simulink subsystem "startNormEcef2Body"  (R2021a)
settings: Solver=VariableStepAuto  StartTime=0.0  StopTime=10.0  RelTol=1e-3
libraries: dspmathops x1, sharedtransform x1
settings Model: Creator=noraw  LastModifiedBy=noraw

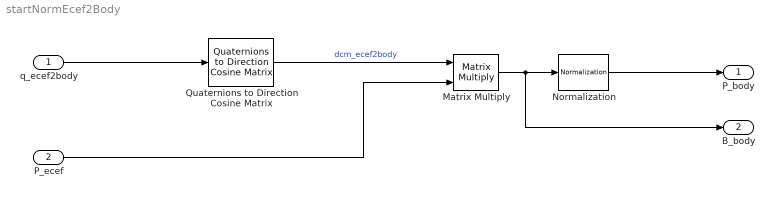
== system startNormEcef2Body ==
  q_ecef2body : Inport  PortDimensions=4
  P_ecef : Inport  Port=2  PortDimensions=3
  Matrix Multiply : Product  Multiplication=Matrix(*)
  Normalization : dspmathops/Normalization  NormType=2-norm  Bias=1e-10  NormOver=Each column  Dimension=1  roundingMode=Floor  overflowMode=off  accumDataTypeStr=Inherit: Same as product output  accumLastDataTypeStr=Inherit: Same as product output  outputDataTypeStr=Inherit: Same as product output  outputMin=[]  outputMax=[]  outputLastDataTypeStr=Inherit: Same as product output
  Quaternions to Direction Cosine Matrix : sharedtransform/Quaternions to  Direction Cosine Matrix  aMode=aMode
      settings: SourceProductBaseCode=AE,PW,DR,MT,UV,VE
  P_body : Outport
  B_body : Outport  Port=2
  wires:
  Normalization/1 -> P_body/1
  Matrix Multiply/1 -> Normalization/1, B_body/1
  Quaternions to Direction Cosine Matrix/1 -> Matrix Multiply/1  "dcm_ecef2body"
  P_ecef/1 -> Matrix Multiply/2
  q_ecef2body/1 -> Quaternions to Direction Cosine Matrix/1
